simulink model "Gestione_Agricola_2023a"  (R2023b)
settings: Solver=VariableStepAuto  StartTime=0.0  StopTime=600  RelTol=1e-3
undefined symbols (not defined in the file or in its folder): ZigBee
libraries: truetime x14, fuzblock x5
settings Model: Creator=giovanni02  LastModifiedBy=francescopaoloseverino

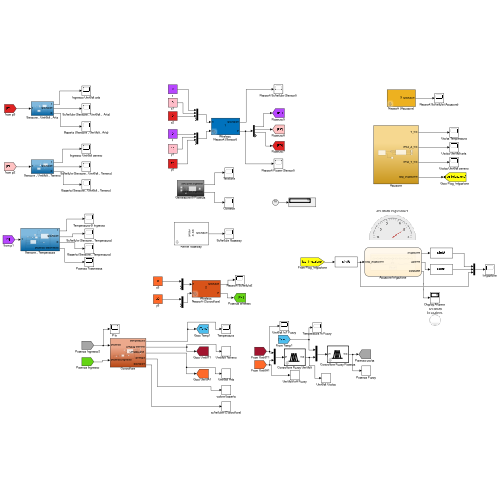
[thumbnail: Simulink's stored preview of the top-level diagram]
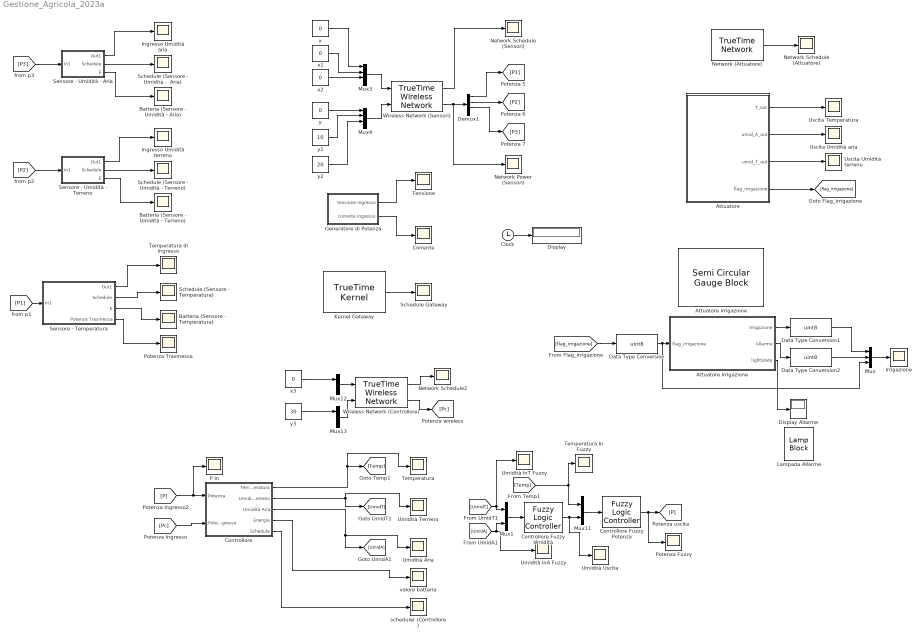
== system Gestione_Agricola_2023a ==
  Attuatore : Subsystem
  Attuatore Irrigazione : Stateflow chart  TreatAsAtomicUnit=on
  Attuatore irrigazione : SemiCircularGaugeBlock  ScaleMax=10  ScaleDirection=Counterclockwise
  Batteria (Sensore - Temperatura) : Scope
  Batteria (Sensore - Umidità - Aria) : Scope
  Batteria (Sensore - Umidità - Terreno) : Scope
  Clock : Clock
  Controllore : Subsystem
  Controllore Fuzzy Potenza : fuzblock/Fuzzy Logic  Controller  FIS='ControlloreFuzzy.fis'  OutputSampleNumber=101  DataType=double  FuzzifiedInputs=off  RuleFiringStrengths=off  RuleOutputs=off  AggregatedOutputs=off  SimulateUsing=Interpreted execution  OutOfRangeInputValueMessage=warning  NoRuleFiredMessage=warning  EmptyOutputFuzzySetMessage=warning
  Controllore Fuzzy Umidità : fuzblock/Fuzzy Logic  Controller  FIS='umidita.fis'  OutputSampleNumber=101  DataType=double  FuzzifiedInputs=off  RuleFiringStrengths=off  RuleOutputs=off  AggregatedOutputs=off  SimulateUsing=Interpreted execution  OutOfRangeInputValueMessage=warning  NoRuleFiredMessage=warning  EmptyOutputFuzzySetMessage=warning
  Corrente : Scope
  Data Type Conversion : DataTypeConversion  OutDataTypeStr=uint8  SaturateOnIntegerOverflow=off  RndMeth=Floor
  Data Type Conversion1 : DataTypeConversion  OutDataTypeStr=uint8  SaturateOnIntegerOverflow=off  RndMeth=Floor
  Data Type Conversion2 : DataTypeConversion  OutDataTypeStr=uint8  SaturateOnIntegerOverflow=off  RndMeth=Floor
  Demux1 : Demux
  Display : Display
  Display Allarme : Display
  Generatore di Potenza : Subsystem
  Ingresso Umidità aria : Scope
  Ingresso Umidità terreno : Scope
  Irrigazione : Scope
  Kernel Gateway : truetime/TrueTime Kernel  sfun=Gateway_init  args=[]  ninputsoutputs=[0 0]  ntriggers=0  trigtype=falling  nwnodenbr=[1 4; 2 4; 3 4]  clockoffsetdrift=[0 0]  schedoutput=on  battery=off  poweroutput=off  label=1: 4\n2: 4\n3: 4
  Lampada Allarme : LampBlock
  Mux : Mux  Inputs=3
  Mux{1,11..13} (4 alike) : Mux  Inputs=2
  Mux3 : Mux
  Mux4 : Mux
  Network (Attuatore) : truetime/TrueTime Network  nwtype=CSMA/CD (Ethernet)  nwnbr=3  nnodes=4  rate=10000000  minsize=512  lossprob=0  seed=0  bandwidths=[0.5 0.5]  slotsize=512  schedule=[1 1 2]  memsize=80000  buftype=Common buffer  overflow=Retransmit  dynSchedule=0  miniSlotSize=0  NIT=0  QSortMode=FIFO  sync=0  irtSchedule=0  nrtLength=0  nodeGraph=0  scheduleoutput=on
  Network Power (Sensori) : Scope
  Network Schedule (Attuatore) : Scope
  Network Schedule (Sensori) : Scope
  Network Schedule2 : Scope
  P In : Scope
  Potenza Fuzzy : Scope
  Potenza Trasmessa : Scope
  Schedule (Sensore - Temperatura) : Scope
  Schedule (Sensore - Umidità -  Aria) : Scope
  Schedule (Sensore - Umidità - Terreno) : Scope
  Schedule Gateway : Scope
  Sensore - Temperatura : Subsystem
  Sensore - Umidità - Aria : Subsystem
  Sensore - Umidità - Terreno : Subsystem
  "Temperatura " : Scope
  Temperatura In Fuzzy : Scope
  Temperatura di ingresso : Scope
  Tensione : Scope
  Umidità Aria : Scope
  Umidità InA Fuzzy : Scope
  Umidità InT Fuzzy : Scope
  Umidità Terreno : Scope
  Umidità Uscita : Scope
  Uscita Temperatura : Scope
  Uscita Umidità aria : Scope
  Uscita Umidità terreno : Scope
  Wireless Network (Controllore) : truetime/TrueTime Wireless  Network  nwtype=802.15.4 (ZigBee)  nwnbr=2  nnodes=4  rate=800000  minsize=272  transpower=20  threshold=-48  use_pathloss_function=default  pathloss=3.5  acktimeout=0.00004  retrylimit=5  error_threshold=0.03  lossprob=0  seed=0  scheduleoutput=on  poweroutput=on
  Wireless Network (Sensori) : truetime/TrueTime Wireless  Network  nwtype=802.15.4 (ZigBee)  nwnbr=1  nnodes=6  rate=800000  minsize=272  transpower=20  threshold=-48  use_pathloss_function=default  pathloss=3.5  acktimeout=0.00004  retrylimit=5  error_threshold=0.03  lossprob=0  seed=0  scheduleoutput=on  poweroutput=on
  scheduler (Controllore) : Scope
  valore batteria : Scope
  x{,1..3} (4 alike) : Constant  Value=0
  y : Constant  Value=0
  y1 : Constant  Value=10
  y2 : Constant  Value=20
  y3 : Constant  Value=30
  wires:
  Kernel Gateway/1 -> Schedule Gateway/1
  Network (Attuatore)/1 -> Network Schedule (Attuatore)/1
  Mux11/1 -> Controllore Fuzzy Potenza/1
  Mux3/1 -> Wireless Network (Sensori)/1
  Mux12/1 -> Wireless Network (Controllore)/1
  y2/1 -> Mux4/3
  Wireless Network (Sensori)/2 -> Demux1/1, Network Power (Sensori)/1
  Wireless Network (Sensori)/1 -> Network Schedule (Sensori)/1
  Clock/1 -> Display/1
  Wireless Network (Controllore)/1 -> Network Schedule2/1
  Mux13/1 -> Wireless Network (Controllore)/2
  Demux1/2 -> [P2]
  Wireless Network (Controllore)/2 -> [Pc]
  [Temp] -> Mux11/1, Temperatura In Fuzzy/1
  x3/1 -> Mux12/1
  Demux1/3 -> [P3]
  [P] -> Controllore/1(Potenza), P In/1
  x/1 -> Mux3/1
  Mux4/1 -> Wireless Network (Sensori)/2
  y1/1 -> Mux4/2
  y3/1 -> Mux13/1
  Controllore Fuzzy Potenza/1 -> Potenza Fuzzy/1, [P]
  y/1 -> Mux4/1
  x2/1 -> Mux3/3
  Demux1/1 -> [P1]
  x1/1 -> Mux3/2
  [P3] -> Sensore - Umidità - Aria/1(In1)
  Sensore - Umidità - Aria/1(Out1) -> Ingresso Umidità aria/1
  Sensore - Umidità - Aria/2(Schedule) -> Schedule (Sensore - Umidità -  Aria)/1
  Sensore - Umidità - Aria/3(E) -> Batteria (Sensore - Umidità - Aria)/1
  [P2] -> Sensore - Umidità - Terreno/1(In1)
  Sensore - Umidità - Terreno/1(Out1) -> Ingresso Umidità terreno/1
  Sensore - Umidità - Terreno/2(Schedule) -> Schedule (Sensore - Umidità - Terreno)/1
  Sensore - Umidità - Terreno/3(E) -> Batteria (Sensore - Umidità - Terreno)/1
  [P1] -> Sensore - Temperatura/1(In1)
  Sensore - Temperatura/1(Out1) -> Temperatura di ingresso/1
  Sensore - Temperatura/2(Schedule) -> Schedule (Sensore - Temperatura)/1
  Sensore - Temperatura/3(E) -> Batteria (Sensore - Temperatura)/1
  Controllore/3("Umidità Aria ") -> [UmidA], Umidità Aria/1
  Controllore/2(Umidità Terreno) -> [UmidT], Umidità Terreno/1
  Controllore/1(Temperatura) -> "Temperatura "/1, [Temp]
  [Pc] -> Controllore/2(Potenza Ingresso)
  Controllore/4(Energia) -> valore batteria/1
  Controllore/5(Schedule) -> scheduler (Controllore)/1
  Data Type Conversion/1 -> Mux/3, Attuatore Irrigazione/1(flag_irrigazione)
  Attuatore Irrigazione/1(Irrigazione) -> Data Type Conversion1/1
  Data Type Conversion1/1 -> Mux/1
  Mux/1 -> Irrigazione/1
  Attuatore Irrigazione/2(Allarme) -> Data Type Conversion2/1
  Data Type Conversion2/1 -> Mux/2
  Attuatore/1(T_out) -> Uscita Temperatura/1
  Attuatore/2(umid_A_out) -> Uscita Umidità aria/1
  Attuatore/3(umid_T_out) -> Uscita Umidità terreno/1
  Attuatore/4(flag_irrigazione) -> [flag_irrigazione]
  [flag_irrigazione] -> Data Type Conversion/1
  Attuatore Irrigazione/3(lightState) -> Display Allarme/1
  [UmidT] -> Mux1/1, Umidità InT Fuzzy/1
  [UmidA] -> Umidità InA Fuzzy/1, Mux1/2
  Mux1/1 -> Controllore Fuzzy Umidità/1
  Controllore Fuzzy Umidità/1 -> Umidità Uscita/1, Mux11/2
  Sensore - Temperatura/4(Potenza Trasmessa) -> Potenza Trasmessa/1
  Generatore di Potenza/1(tensione Ingresso) -> Tensione/1
  Generatore di Potenza/2(corrente Ingresso) -> Corrente/1

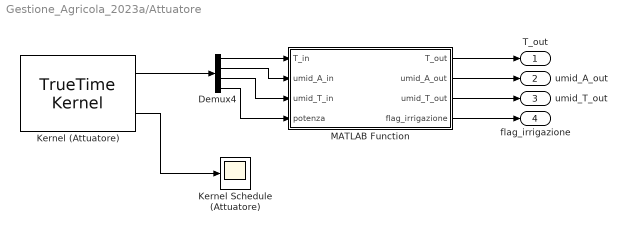
== system Gestione_Agricola_2023a/Attuatore ==
  Demux4 : Demux
  Kernel (Attuatore) : truetime/TrueTime Kernel  sfun=Attuatore_init  args=[]  ninputsoutputs=[0 4]  ntriggers=0  trigtype=falling  nwnodenbr=[3 1]  clockoffsetdrift=[0 0]  schedoutput=on  battery=off  poweroutput=off  label=3: 1
  Kernel Schedule (Attuatore) : Scope
  MATLAB Function : MATLAB Function  TreatAsAtomicUnit=on
  T_out : Outport
  umid_A_out : Outport  Port=2
  umid_T_out : Outport  Port=3
  flag_irrigazione : Outport  Port=4
  wires:
  Demux4/1 -> MATLAB Function/1(T_in)
  Demux4/2 -> MATLAB Function/2(umid_A_in)
  Demux4/3 -> MATLAB Function/3(umid_T_in)
  Demux4/4 -> MATLAB Function/4(potenza)
  Kernel (Attuatore)/2 -> Kernel Schedule (Attuatore)/1
  Kernel (Attuatore)/1 -> Demux4/1
  MATLAB Function/1(T_out) -> T_out/1
  MATLAB Function/2(umid_A_out) -> umid_A_out/1
  MATLAB Function/3(umid_T_out) -> umid_T_out/1
  MATLAB Function/4(flag_irrigazione) -> flag_irrigazione/1

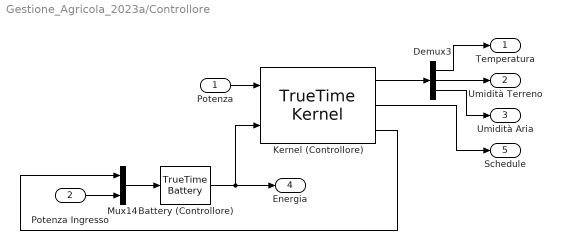
== system Gestione_Agricola_2023a/Controllore ==
  Potenza : Inport
  Potenza Ingresso : Inport  Port=2
  Battery (Controllore) : truetime/TrueTime Battery  energy=50
  Demux3 : Demux  Outputs=3
  Kernel (Controllore) : truetime/TrueTime Kernel  sfun=Controllore_init  args=[]  ninputsoutputs=[1 3]  ntriggers=0  trigtype=falling  nwnodenbr=[2 2]  clockoffsetdrift=[0 0]  schedoutput=on  battery=on  poweroutput=on  label=2: 2
  Mux14 : Mux  Inputs=2
  Temperatura : Outport
  Umidità Terreno : Outport  Port=2
  "Umidità Aria " : Outport  Port=3
  Energia : Outport  Port=4
  Schedule : Outport  Port=5
  wires:
  Potenza Ingresso/1 -> Mux14/2
  Mux14/1 -> Battery (Controllore)/1
  Kernel (Controllore)/2 -> Schedule/1
  Demux3/3 -> "Umidità Aria "/1
  Demux3/2 -> Umidità Terreno/1
  Potenza/1 -> Kernel (Controllore)/1
  Kernel (Controllore)/3 -> Mux14/1
  Demux3/1 -> Temperatura/1
  Kernel (Controllore)/1 -> Demux3/1
  Battery (Controllore)/1 -> Energia/1, Kernel (Controllore)/2

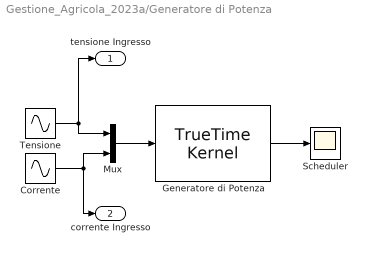
== system Gestione_Agricola_2023a/Generatore di Potenza ==
  Corrente : Sin  Amplitude=0.05  SampleTime=0
  Generatore di Potenza : truetime/TrueTime Kernel  sfun=Generatore_di_potenza_init  args=[]  ninputsoutputs=[2 0]  ntriggers=0  trigtype=falling  nwnodenbr=[1 5]  clockoffsetdrift=[0 0]  schedoutput=on  battery=off  poweroutput=off  label=1: 5
  Mux : Mux  Inputs=2
  Scheduler : Scope
  Tensione : Sin  Amplitude=18  Phase=pi / 2  SampleTime=0
  tensione Ingresso : Outport
  corrente Ingresso : Outport  Port=2
  wires:
  Mux/1 -> Generatore di Potenza/1
  Generatore di Potenza/1 -> Scheduler/1
  Tensione/1 -> tensione Ingresso/1, Mux/1
  Corrente/1 -> corrente Ingresso/1, Mux/2

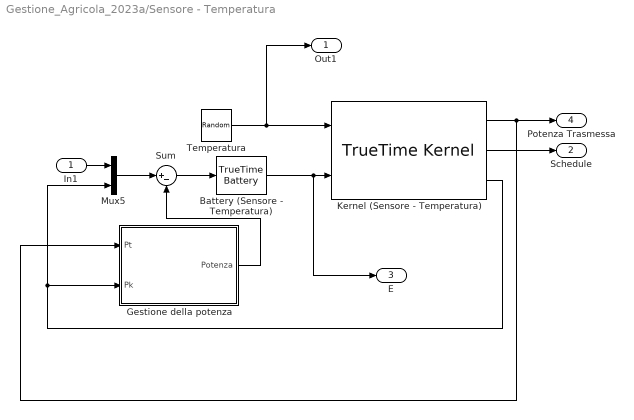
== system Gestione_Agricola_2023a/Sensore - Temperatura ==
  In1 : Inport
  "Battery (Sensore - Temperatura) " : truetime/TrueTime Battery  energy=10
  Gestione della potenza : Subsystem
  Kernel (Sensore - Temperatura) : truetime/TrueTime Kernel  sfun=Sensore_temperatura_init  args=[]  ninputsoutputs=[1 1]  ntriggers=0  trigtype=falling  nwnodenbr=[1 1]  clockoffsetdrift=[0 0]  schedoutput=on  battery=on  poweroutput=on  label=1: 1
  Mux5 : Mux  Inputs=2
  Sum : Sum  Inputs=|+-
  Temperatura : UniformRandomNumber  Minimum=10  Maximum=40  Seed=5  SampleTime=1
  Out1 : Outport
  Schedule : Outport  Port=2
  E : Outport  Port=3
  Potenza Trasmessa : Outport  Port=4
  wires:
  Temperatura/1 -> Out1/1, Kernel (Sensore - Temperatura)/1
  Kernel (Sensore - Temperatura)/2 -> Schedule/1
  "Battery (Sensore - Temperatura) "/1 -> Kernel (Sensore - Temperatura)/2, E/1
  In1/1 -> Mux5/1
  Mux5/1 -> Sum/1
  Sum/1 -> "Battery (Sensore - Temperatura) "/1
  Gestione della potenza/1(Potenza) -> Sum/2
  Kernel (Sensore - Temperatura)/3 -> Mux5/2, Gestione della potenza/2(Pk)
  Kernel (Sensore - Temperatura)/1 -> Gestione della potenza/1(Pt), Potenza Trasmessa/1

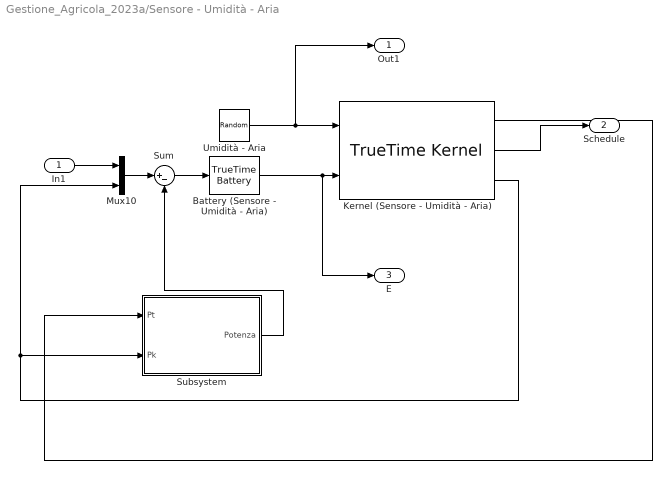
== system Gestione_Agricola_2023a/Sensore - Umidità - Aria ==
  In1 : Inport
  Battery (Sensore - Umidità - Aria) : truetime/TrueTime Battery  energy=10
  Kernel (Sensore - Umidità - Aria) : truetime/TrueTime Kernel  sfun=Sensore_umidita_aria_init  args=[]  ninputsoutputs=[1 1]  ntriggers=0  trigtype=falling  nwnodenbr=[1 3]  clockoffsetdrift=[0 0]  schedoutput=on  battery=on  poweroutput=on  label=1: 3
  Mux10 : Mux  Inputs=2
  Subsystem : Subsystem
  Sum : Sum  Inputs=|+-
  Umidità - Aria : UniformRandomNumber  Minimum=30  Maximum=90  Seed=5  SampleTime=1
  Out1 : Outport
  Schedule : Outport  Port=2
  E : Outport  Port=3
  wires:
  Umidità - Aria/1 -> Out1/1, Kernel (Sensore - Umidità - Aria)/1
  In1/1 -> Mux10/1
  Battery (Sensore - Umidità - Aria)/1 -> E/1, Kernel (Sensore - Umidità - Aria)/2
  Kernel (Sensore - Umidità - Aria)/2 -> Schedule/1
  Kernel (Sensore - Umidità - Aria)/3 -> Subsystem/2(Pk), Mux10/2
  Mux10/1 -> Sum/1
  Sum/1 -> Battery (Sensore - Umidità - Aria)/1
  Subsystem/1(Potenza) -> Sum/2
  Kernel (Sensore - Umidità - Aria)/1 -> Subsystem/1(Pt)

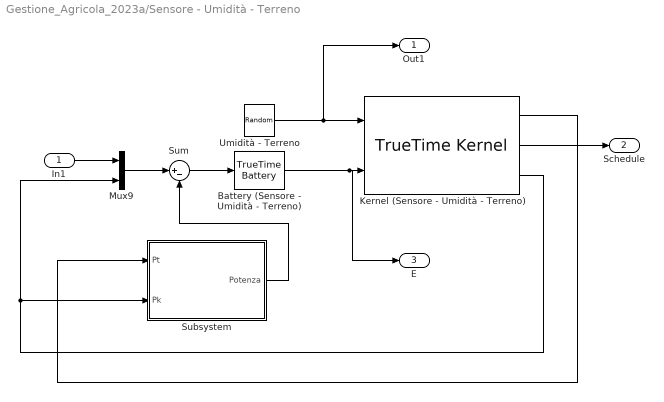
== system Gestione_Agricola_2023a/Sensore - Umidità - Terreno ==
  In1 : Inport
  "Battery (Sensore - Umidità - Terreno) " : truetime/TrueTime Battery  energy=10
  Kernel (Sensore - Umidità - Terreno) : truetime/TrueTime Kernel  sfun=Sensore_umidita_terreno_init  args=[]  ninputsoutputs=[1 1]  ntriggers=0  trigtype=falling  nwnodenbr=[1 2]  clockoffsetdrift=[0 0]  schedoutput=on  battery=on  poweroutput=on  label=1: 2
  Mux9 : Mux  Inputs=2
  Subsystem : Subsystem
  Sum : Sum  Inputs=|+-
  Umidità - Terreno : UniformRandomNumber  Minimum=30  Maximum=90  Seed=5  SampleTime=1
  Out1 : Outport
  Schedule : Outport  Port=2
  E : Outport  Port=3
  wires:
  Kernel (Sensore - Umidità - Terreno)/2 -> Schedule/1
  Umidità - Terreno/1 -> Out1/1, Kernel (Sensore - Umidità - Terreno)/1
  In1/1 -> Mux9/1
  "Battery (Sensore - Umidità - Terreno) "/1 -> E/1, Kernel (Sensore - Umidità - Terreno)/2
  Kernel (Sensore - Umidità - Terreno)/3 -> Subsystem/2(Pk), Mux9/2
  Mux9/1 -> Sum/1
  Sum/1 -> "Battery (Sensore - Umidità - Terreno) "/1
  Subsystem/1(Potenza) -> Sum/2
  Kernel (Sensore - Umidità - Terreno)/1 -> Subsystem/1(Pt)

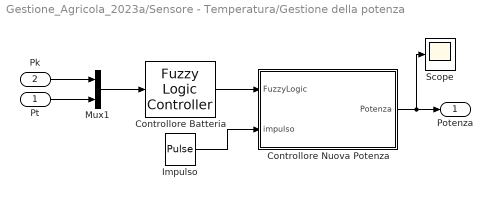
== system Gestione_Agricola_2023a/Sensore - Temperatura/Gestione della potenza ==
  Pt : Inport
  Pk : Inport  Port=2
  Controllore Batteria : fuzblock/Fuzzy Logic  Controller  FIS='battery.fis'  OutputSampleNumber=101  DataType=double  FuzzifiedInputs=off  RuleFiringStrengths=off  RuleOutputs=off  AggregatedOutputs=off  SimulateUsing=Interpreted execution  OutOfRangeInputValueMessage=warning  NoRuleFiredMessage=warning  EmptyOutputFuzzySetMessage=warning
  Controllore Nuova Potenza : MATLAB Function  TreatAsAtomicUnit=on
  Impulso : DiscretePulseGenerator  PulseType=Time based  Amplitude=0.1  Period=1  PulseWidth=5
  Mux1 : Mux  Inputs=2
  Scope : Scope
  Potenza : Outport
  wires:
  Controllore Batteria/1 -> Controllore Nuova Potenza/1(FuzzyLogic)
  Mux1/1 -> Controllore Batteria/1
  Impulso/1 -> Controllore Nuova Potenza/2(impulso)
  Controllore Nuova Potenza/1(Potenza) -> Scope/1, Potenza/1
  Pk/1 -> Mux1/1
  Pt/1 -> Mux1/2

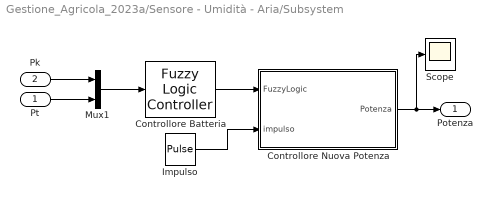
== system Gestione_Agricola_2023a/Sensore - Umidità - Aria/Subsystem ==
  Pt : Inport
  Pk : Inport  Port=2
  Controllore Batteria : fuzblock/Fuzzy Logic  Controller  FIS='battery.fis'  OutputSampleNumber=101  DataType=double  FuzzifiedInputs=off  RuleFiringStrengths=off  RuleOutputs=off  AggregatedOutputs=off  SimulateUsing=Interpreted execution  OutOfRangeInputValueMessage=warning  NoRuleFiredMessage=warning  EmptyOutputFuzzySetMessage=warning
  Controllore Nuova Potenza : MATLAB Function  TreatAsAtomicUnit=on
  Impulso : DiscretePulseGenerator  PulseType=Time based  Amplitude=0.1  Period=1  PulseWidth=5
  Mux1 : Mux  Inputs=2
  Scope : Scope
  Potenza : Outport
  wires:
  Controllore Batteria/1 -> Controllore Nuova Potenza/1(FuzzyLogic)
  Mux1/1 -> Controllore Batteria/1
  Impulso/1 -> Controllore Nuova Potenza/2(impulso)
  Controllore Nuova Potenza/1(Potenza) -> Scope/1, Potenza/1
  Pk/1 -> Mux1/1
  Pt/1 -> Mux1/2

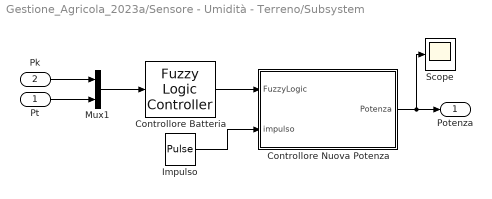
== system Gestione_Agricola_2023a/Sensore - Umidità - Terreno/Subsystem ==
  Pt : Inport
  Pk : Inport  Port=2
  Controllore Batteria : fuzblock/Fuzzy Logic  Controller  FIS='battery.fis'  OutputSampleNumber=101  DataType=double  FuzzifiedInputs=off  RuleFiringStrengths=off  RuleOutputs=off  AggregatedOutputs=off  SimulateUsing=Interpreted execution  OutOfRangeInputValueMessage=warning  NoRuleFiredMessage=warning  EmptyOutputFuzzySetMessage=warning
  Controllore Nuova Potenza : MATLAB Function  TreatAsAtomicUnit=on
  Impulso : DiscretePulseGenerator  PulseType=Time based  Amplitude=0.1  Period=1  PulseWidth=5
  Mux1 : Mux  Inputs=2
  Scope : Scope
  Potenza : Outport
  wires:
  Controllore Batteria/1 -> Controllore Nuova Potenza/1(FuzzyLogic)
  Mux1/1 -> Controllore Batteria/1
  Impulso/1 -> Controllore Nuova Potenza/2(impulso)
  Controllore Nuova Potenza/1(Potenza) -> Scope/1, Potenza/1
  Pk/1 -> Mux1/1
  Pt/1 -> Mux1/2

== matlab function Gestione_Agricola_2023a/Sensore - Umidità - Terreno/Subsystem/Controllore Nuova Potenza ==
  data: FuzzyLogic input; Potenza output; impulso input
function Potenza = fcn(FuzzyLogic, impulso)

if FuzzyLogic >= 0.06
    Potenza = FuzzyLogic * impulso * 1; %MAX 0.09
elseif FuzzyLogic < 0.06 && FuzzyLogic > 0.04
    Potenza = FuzzyLogic * impulso * 1.8; %MAX 0.09
else
    Potenza = FuzzyLogic * impulso * 3; % MAX 0.09
end

== stateflow chart Gestione_Agricola_2023a/Attuatore Irrigazione ==
  state SistemaGestioneIrrigazioneAllarme
    state IrrigazioneOnOff [parallel]
      settings: executionOrder=1
      state Stato0
        entry: Irrigazione = uint8(0);
        Allarme = uint8(0);
        switchPos = false;
      state Stato1
        entry: Irrigazione = uint8(1);
        Allarme = uint8(0);
        switchPos = false;
      state Stato2
        entry: Irrigazione = uint8(2);
        Allarme = uint8(0);
        switchPos = false;
      state Stato3
        entry: Irrigazione = uint8(3);
        Allarme = uint8(0);
        switchPos = false;
      state Stato4
        entry: Irrigazione = uint8(4);
        Allarme = uint8(0);
        switchPos = false;
      state Stato5
        entry: Irrigazione = uint8(5);
        Allarme = uint8(0);
        switchPos = false;
      state Stato6
        entry: Irrigazione = uint8(6);
        Allarme = uint8(0);
        switchPos = false;
      state Stato7
        entry: Irrigazione = uint8(7);
        Allarme = uint8(0);
        switchPos = false;
      state Stato8
        entry: Irrigazione = uint8(8);
        Allarme = uint8(0);
        switchPos = false;
      state Stato9
        entry: Irrigazione = uint8(9);
        Allarme = uint8(0);
        switchPos = false;
      state Stato10
        entry: Irrigazione = uint8(10);
        Allarme = uint8(0);
        switchPos = false;
      state Allarme
        entry: Allarme = uint8(1);
        Irrigazione = uint8(0);
        switchPos = true;
      Stato5 -> Stato5 [order 2] : [duration(flag_irrigazione == 1) > 0.5]
      Stato9 -> Stato9 [order 2] : [duration(flag_irrigazione == 1) > 0.5]
      Stato6 -> Stato6 [order 2] : [duration(flag_irrigazione == 1) > 0.5]
      Stato3 -> Stato3 [order 2] : [duration(flag_irrigazione == 1) > 0.5]
      Stato10 -> Stato10 [order 2] : [duration(flag_irrigazione == 1) > 0.5]
      Stato0 -> Stato0 [order 2] : [duration(flag_irrigazione == 1) > 0.5]
      Stato1 -> Stato1 [order 2] : [duration(flag_irrigazione == 1) > 0.5]
      Stato2 -> Stato2 [order 3] : [duration(flag_irrigazione == 1) > 0.5]
      Stato4 -> Stato4 [order 2] : [duration(flag_irrigazione == 1) > 0.5]
      Stato7 -> Stato7 [order 2] : [duration(flag_irrigazione == 1) > 0.5]
      Stato8 -> Stato8 [order 2] : [duration(flag_irrigazione == 1) > 0.5]
      Stato4 -> Stato5 [order 1] : [duration(flag_irrigazione == 2) > 0.5]
      Stato5 -> Stato6 [order 1] : [duration(flag_irrigazione == 2) > 0.5]
      Stato6 -> Stato7 [order 1] : [duration(flag_irrigazione == 2) > 0.5]
      Stato2 -> Stato3 [order 1] : [duration(flag_irrigazione == 2) > 0.5]
      Stato3 -> Stato4 [order 1] : [duration(flag_irrigazione == 2) > 0.5]
      Stato1 -> Stato2 [order 1] : [duration(flag_irrigazione == 2) > 0.5]
      Stato0 -> Stato1 [order 1] : [duration(flag_irrigazione == 2) > 0.5]
      Stato7 -> Stato8 [order 1] : [duration(flag_irrigazione == 2) > 0.5]
      Stato8 -> Stato9 [order 1] : [duration(flag_irrigazione == 2) > 0.5]
      Stato9 -> Stato10 [order 1] : [duration(flag_irrigazione == 2) > 0.5]
      Stato3 -> Stato2 [order 3] : [duration(flag_irrigazione == 0) > 0.5]
      Stato4 -> Stato3 [order 3] : [duration(flag_irrigazione == 0) > 0.5]
      Stato7 -> Stato6 [order 3] : [duration(flag_irrigazione == 0) > 0.5]
      Stato5 -> Stato4 [order 3] : [duration(flag_irrigazione == 0) > 0.5]
      Stato8 -> Stato7 [order 3] : [duration(flag_irrigazione == 0) > 0.5]
      Stato1 -> Stato0 [order 3] : [duration(flag_irrigazione == 0) > 0.5]
      Stato6 -> Stato5 [order 3] : [duration(flag_irrigazione == 0) > 0.5]
      Stato2 -> Stato1 [order 2] : [duration(flag_irrigazione == 0) > 0.5]
      Stato9 -> Stato8 [order 3] : [duration(flag_irrigazione == 0) > 0.5]
      Stato10 -> Stato9 [order 1] : [duration(flag_irrigazione == 0) > 0.5]
      Stato0 -> Allarme [order 3] : [duration(flag_irrigazione == 0) > 0.5]
      (default) -> Stato5
      Allarme -> Stato5 [order 2] : [duration(flag_irrigazione == 1) > 0.5]
      Stato10 -> Allarme [order 3] : [duration(flag_irrigazione == 2) > 0.5]
      Allarme -> Allarme [order 3] : [duration(flag_irrigazione == 2) > 0.5]
      Allarme -> Allarme [order 1] : [duration(flag_irrigazione == 0) > 0.5]
    state LampadaAllarme [parallel]
      settings: executionOrder=2
      state OFF
        entry:
        lightState=0;
      state ON
        entry:
        lightState=1;
      (default) -> OFF
      OFF -> ON : [switchPos==true]
      ON -> OFF [order 1] : [switchPos==false]
      ON -> OFF [order 2] : after(3,sec)
  data: flag_irrigazione input uint8; Irrigazione output uint8; Allarme output uint8; lightState output uint8; switchPos local boolean

== matlab function Gestione_Agricola_2023a/Sensore - Temperatura/Gestione della potenza/Controllore Nuova Potenza ==
  data: FuzzyLogic input; Potenza output; impulso input
function Potenza = fcn(FuzzyLogic, impulso)

if FuzzyLogic >= 0.06
    Potenza = FuzzyLogic * impulso * 1; %MAX 0.09
elseif FuzzyLogic < 0.06 && FuzzyLogic > 0.04
    Potenza = FuzzyLogic * impulso * 1.8; %MAX 0.09
else
    Potenza = FuzzyLogic * impulso * 3; % MAX 0.09
end

== matlab function Gestione_Agricola_2023a/Sensore - Umidità - Aria/Subsystem/Controllore Nuova Potenza ==
  data: FuzzyLogic input; Potenza output; impulso input
function Potenza = fcn(FuzzyLogic, impulso)

if FuzzyLogic >= 0.06
    Potenza = FuzzyLogic * impulso * 1; %MAX 0.09
elseif FuzzyLogic < 0.06 && FuzzyLogic > 0.04
    Potenza = FuzzyLogic * impulso * 1.8; %MAX 0.09
else
    Potenza = FuzzyLogic * impulso * 3; % MAX 0.09
end

== matlab function Gestione_Agricola_2023a/Attuatore/MATLAB Function ==
  data: T_in input; T_out output; umid_A_in input; umid_T_in input; potenza input; umid_A_out output; umid_T_out output; flag_irrigazione output
function [T_out, umid_A_out, umid_T_out, flag_irrigazione] = fcn(T_in, umid_A_in, umid_T_in, potenza)
umid_A_out = umid_A_in;
umid_T_out = umid_T_in;
T_out = T_in;
flag_irrigazione = 1;

if potenza >= 6.5
    while umid_A_out > 55.5 && umid_T_out > 52.5
        umid_A_out = umid_A_out - potenza * 1.5;
        umid_T_out = umid_T_out - potenza * 1.5;
        %disp('valore umidita terreno uscita:');
        %disp(umid_T_out);
    end

    if T_in >= 25.5
        while T_out > 20
            T_out = T_out - potenza * 1.5;
            %disp('valore temperatura uscita:');
            %disp(T_out);
        end
    end
    

    flag_irrigazione = 0; %diminuisci

elseif potenza >= 5 && potenza < 6.5
    if T_in >= 25.5
        while T_out > 20
            T_out = T_out - potenza * 1.5;
            %disp('valore temperatura 2 uscita:');
            %disp(T_out);
        end
    end

    if umid_T_in > 38
        umid_T_out = umid_T_out - potenza;
    end

    if umid_A_in > 35
        umid_A_out = umid_A_out - potenza;
    end

    flag_irrigazione = 1; %mantieni

elseif potenza < 5
    umid_A_out = umid_A_out + potenza;
    umid_T_out = umid_T_out + potenza;

    if T_in <= 15
        T_out = T_out + potenza * 1.5;
    end

    flag_irrigazione = 2; %aumenta
    %disp(flag_irrigazione);
end
